simulink model "predicteur_de_smith"  (R2017a)
settings: Solver=ode45  StartTime=0.0  StopTime=5.0  MaxStep=0.01  RelTol=1e-3  EnableMultiTasking=on
settings Model: ExtModeAutoUpdateStatusClock=off  Creator=jacques  LastModifiedBy=PC
settings DataIOCC: LimitDataPoints=on  SaveFormat=Array  SignalLoggingSaveFormat=ModelDataLogs
settings OptimizationCC: ExpressionDepthLimit=2147483647  InitFltsAndDblsToZero=on  LifeSpan=inf
settings DebuggingCC: UnderspecifiedInitializationDetection=Classic  MergeDetectMultiDrivingBlocksExec=none  SolverPrmCheckMsg=warning  FcnCallInpInsideContextMsg=warning  StateNameClashWarn=warning  SFUnexpectedBacktrackingDiag=warning  SFNoUnconditionalDefaultTransitionDiag=warning  SFExecutionAtInitializationDiag=none
settings HardwareCC: ProdBitPerPointer=32  ProdBitPerSizeT=32  ProdBitPerPtrDiffT=32  ProdLargestAtomicFloat=None  ProdIntDivRoundTo=Undefined  ProdEndianess=Unspecified  ProdWordSize=32  ProdHWDeviceType=32-bit Generic
settings ModelReferenceCC: PropagateSignalLabelsOutOfModel=off
settings GRTTargetCC: TargetLangStandard=C89/C90 (ANSI)  GeneratePreprocessorConditionals=Disable all  CombineOutputUpdateFcns=off  GRTInterface=on
settings ConfigComp: CovMetricSettings=dw  CovHtmlReporting=on  CovSaveCumulativeToWorkspaceVar=on  CovSaveSingleToWorkspaceVar=on  CovExternalEMLEnable=off

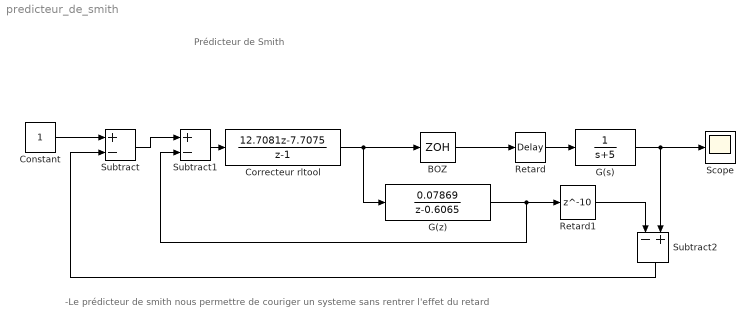
== system predicteur_de_smith ==
  note: -Le prédicteur de smith nous permettre de couriger un systeme sans rentrer l'effet du retard
  note: Prédicteur de Smith
  BOZ : ZeroOrderHold  SampleTime=0.1
  Constant : Constant
  Correcteur rltool : DiscreteTransferFcn  Numerator="[12.7081   -7.7075]"  Denominator=[1 -1]  SampleTime=0.1
  G(s) : TransferFcn  Denominator=[1 5]
  G(z) : DiscreteTransferFcn  Numerator=[0.07869]  Denominator=[1 -0.6065]  SampleTime=0.1
  Retard : TransportDelay
  Retard1 : Delay  DelayLength=10  InputProcessing=Inherited  SampleTime=0.1
  Scope : Scope
  Subtract : Sum  Inputs=+-
  Subtract1 : Sum  Inputs=+-
  Subtract2 : Sum  Inputs=-+
  wires:
  Constant/1 -> Subtract/1
  Subtract/1 -> Subtract1/1
  Correcteur rltool/1 -> BOZ/1, G(z)/1
  BOZ/1 -> Retard/1
  Retard/1 -> G(s)/1
  G(s)/1 -> Scope/1, Subtract2/2
  Subtract1/1 -> Correcteur rltool/1
  G(z)/1 -> Subtract1/2, Retard1/1
  Retard1/1 -> Subtract2/1
  Subtract2/1 -> Subtract/2
